simulink model "MATLAB_TEST"  (R2019b)
settings: Solver=FixedStepDiscrete  StartTime=0  StopTime=50  FixedStep=0.0025  RelTol=1e-3
undefined symbols (not defined in the file): BCM_COM_PROC_P20, BCM_COM_PROC_P20_SFW_R2018b, BCM_COM_PROC_P2_5, BCM_COM_PROC_P2_5_SFW_R2018b, BCM_COM_PROC_P5, BCM_COM_PROC_P5_SFW_R2018b, BCMA_ACCU_PT_Conf_Flt, BCMA_ACCU_PT_Unconf_Flt, BCMA_Antiskid_Off_Sanction, BCMA_Avionics_Conf_Flt, BCMA_BCM_CCDL_Conf_Flt, BCMA_BCM_CCDL_Unconf_Flt, BCMA_BCM_DBCU_INHIBITION_Conf_Flt, BCMA_BCM_DBCU_INHIBITION_Unconf_Flt, BCMA_BCP_ALT_Disp_Sw_Conf_Flt, BCMA_BCP_ALT_Disp_Sw_Unconf_Flt, BCMA_BCP_ALT_SW_ON_CMD_Conf_Flt, BCMA_BCP_ALT_SW_ON_CMD_Unconf_Flt, BCMA_BCP_PARK_OFF_SW_CMD_Conf_Flt, BCMA_BCP_PARK_OFF_SW_CMD_Unconf_Flt, BCMA_CF_BSELV_JCL, BCMA_CF_BSELV_JOP, BCMA_CF_BSELV_OC, BCMA_CF_BSELV_SC, BCMA_CF_LH_SV_JCL, BCMA_CF_LH_SV_JOP, BCMA_CF_LH_SV_OC, BCMA_CF_LH_SV_SC, BCMA_CF_PARK_BRK, BCMA_CF_RESIDUAL_PRESS, BCMA_CF_RH_SV_JCL, BCMA_CF_RH_SV_JOP, BCMA_CF_RH_SV_OC, BCMA_CF_RH_SV_SC, BCMA_CF_SELV_JCL, BCMA_CF_SELV_JOP, BCMA_CF_SELV_OC, BCMA_CF_SELV_SC, BCMA_CF_SV_DRIFT, BCMA_DBCU_ALT_MODE_Conf_Flt, BCMA_DBCU_ALT_MODE_Unconf_Flt, BCMA_DBCU_BRK_ORDER_FAIL_Conf_Flt, BCMA_DBCU_BRK_ORDER_FAIL_Unconf_Flt, BCMA_DBCU_Conf_Flt, BCMA_DBCU_DISPATCH_SW_ON_Conf_Flt, BCMA_DBCU_DISPATCH_SW_ON_Unconf_Flt, BCMA_DBCU_FAILED_Conf_Flt, BCMA_DBCU_FAILED_Unconf_Flt, BCMA_DFCS1_Capsule_Validity, BCMA_DFCS1_Label202_Corrupted, BCMA_DFCS1_Label202_Not_Refreshed, BCMA_DFCS1_Label204_Corrupted, BCMA_DFCS1_Label204_Not_Refreshed, BCMA_DFCS1_Label205_Corrupted, BCMA_DFCS1_Label205_Not_Refreshed, BCMA_DFCS1_Label206_Corrupted, BCMA_DFCS1_Label206_Not_Refreshed, BCMA_DFCS1_Label207_Corrupted, BCMA_DFCS1_Label207_Not_Refreshed, BCMA_DFCS3_Capsule_Validity ... (+762)
libraries: simulink x73, lib_MBD_Control x5
(part 4 of 16)

== system MATLAB_TEST/AVIONICS/Brake_Control_Module_Side_A/BCSA Controller CP/BCM Config Computation ==
  note: 0 = OPEN
      | 1 = Ground
      |
      | According to BCM_ETS_REQ_0134:
      | PIN PROG 1 PIN PROG 2 CONFIG
      | Open Open A
      | Open Ground B
      | OTHER Invalid
  PINPROG_BCM_1 : Inport
  PINPROG_BCM_2 : Inport  Port=2
  Compare To Constant : simulink/Logic and Bit Operations/Compare To Constant  relop===  const=1  OutDataTypeStr=boolean
  Compare To Zero2 : simulink/Logic and Bit Operations/Compare To Zero  relop===  OutDataTypeStr=boolean
  Compare To Zero3 : simulink/Logic and Bit Operations/Compare To Zero  relop===  OutDataTypeStr=boolean
  Constant : Constant  Value=0  OutDataTypeStr=int32
  Constant1 : Constant  OutDataTypeStr=int32
  Constant2 : Constant  Value=2  OutDataTypeStr=int32
  Logical Operator : Logic  AllPortsSameDT=off  OutDataTypeStr=boolean
  Logical Operator1 : Logic  AllPortsSameDT=off  OutDataTypeStr=boolean
  Switch : Switch  Criteria=u2 > Threshold
  Switch1 : Switch  Criteria=u2 > Threshold
  BCM_Config : Outport  VectorParamsAs1DForOutWhenUnconnected=off
  wires:
  PINPROG_BCM_2/1 -> Compare To Constant/1, Compare To Zero3/1
  PINPROG_BCM_1/1 -> Compare To Zero2/1
  Compare To Zero2/1 -> Logical Operator1/1, Logical Operator/1
  Compare To Zero3/1 -> Logical Operator/2
  Compare To Constant/1 -> Logical Operator1/2
  Logical Operator/1 -> Switch/2
  Constant/1 -> Switch/1
  Logical Operator1/1 -> Switch1/2
  Switch1/1 -> Switch/3
  Constant1/1 -> Switch1/1
  Constant2/1 -> Switch1/3
  Switch/1 -> BCM_Config/1
